simulink model "mariner_simtr"  (R2018b)
settings: Solver=FixedStepAuto  StartTime=0.0  StopTime=600  FixedStep=0.1  RelTol=1e-3
libraries: neural x211, simulink x2
(part 6 of 10)

== system mariner_simtr/NN transform (No normalization)/Layer 4/Delays 1 ==
  "p{4}" : Inport  PortDimensions=24
      mask Display: e = 0.06;c1 = [120 230 180]/255;c2 = ([120 230 180]+0)/(256+128);c3 = ([120 230 180]+128)/(256+128);patch([0 1 1 0],[0 0 1 1],c1);patch([0 1 1 1-e 1-e 0+e],[0 0 1 1-e 0+e 0+e],c2);patch([0 0 1 1-e 0+e 0+e],[0 1 1 1-e 1-e 0+e],c3);plot([0 1 1 0 0],[0 0 1 1 0]);
  mux : Mux  Inputs=1
      mask Display: e = 0.06;c1 = [120 150 230]/255;c2 = ([120 150 230]+0)/383;c3 = ([120 150 230]+128)/383;patch([0 1 1 0],[0 0 1 1],c1);patch([0 1 1 1-e 1-e 0+e],[0 0 1 1-e 0+e 0+e],c2);patch([0 0 1 1-e 0+e 0+e],[0 1 1 1-e 1-e 0+e],c3);plot([0 1 1 0 0],[0 0 1 1 0]);disp('Mux')
  "pd{4,3}" : Outport
      mask Display: e = 0.06;c1 = [120 230 180]/255;c2 = ([120 230 180]+0)/(256+128);c3 = ([120 230 180]+128)/(256+128);patch([0 1 1 0],[0 0 1 1],c1);patch([0 1 1 1-e 1-e 0+e],[0 0 1 1-e 0+e 0+e],c2);patch([0 0 1 1-e 0+e 0+e],[0 1 1 1-e 1-e 0+e],c3);plot([0 1 1 0 0],[0 0 1 1 0]);
  wires:
  mux/1 -> "pd{4,3}"/1
  "p{4}"/1 -> mux/1

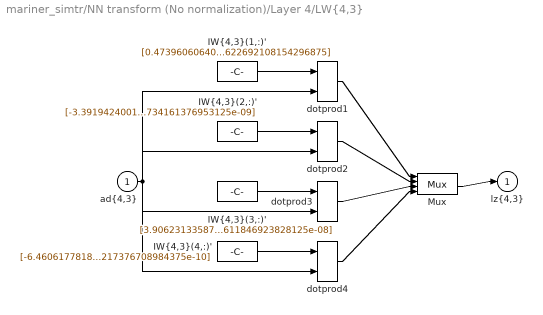
== system mariner_simtr/NN transform (No normalization)/Layer 4/LW{4,3} ==
  "ad{4,3}" : Inport  PortDimensions=24
      mask Display: e = 0.06;c1 = [120 230 180]/255;c2 = ([120 230 180]+0)/(256+128);c3 = ([120 230 180]+128)/(256+128);patch([0 1 1 0],[0 0 1 1],c1);patch([0 1 1 1-e 1-e 0+e],[0 0 1 1-e 0+e 0+e],c2);patch([0 0 1 1-e 0+e 0+e],[0 1 1 1-e 1-e 0+e],c3);plot([0 1 1 0 0],[0 0 1 1 0]);
  "IW{4,3}(1,:)'" : Constant  Value=[0.47396060640014059384128586316364817321300506591796875;0;0;0;0;0.23418587838913584864286576703307218849658966064453125;0.1300136310990274990384563125189743004739284515380859375;0.5442556933540909636093374501797370612621307373046875;0;0;0.1497209490422759803340824191764113493263721466064453125;0.32946160549255931737633318334701471030712127685546875;0;0.58508220152901879718143618447356857359409332275390625;0;0;0.52760521849978292419081071784603409469127655029296875;0;0.4427234693408463872543734396458603441715240478515625;0;0.239017941354947638377126395425875671207904815673828125;0;0;0.342933854164539642095377303121495060622692108154296875]
      mask Display: e = 0.06;c1 = [120 150 230]/255;c2 = ([120 150 230]+0)/383;c3 = ([120 150 230]+128)/383;patch([0 1 1 0],[0 0 1 1],c1);patch([0 1 1 1-e 1-e 0+e],[0 0 1 1-e 0+e 0+e],c2);patch([0 0 1 1-e 0+e 0+e],[0 1 1 1-e 1-e 0+e],c3);plot([0 1 1 0 0],[0 0 1 1 0]);disp('weights');
  "IW{4,3}(2,:)'" : Constant  Value=[-3.391942400136792629749466325699176760810615860464167781174182891845703125e-09;0;0;0;0;-1.6759725826658646329116917372587143575390911109934677369892597198486328125e-09;-9.30453566444665859480412774891629201778897595431772060692310333251953125e-10;-3.89501638174218884460996254154134532665665346939931623637676239013671875e-09;0;0;-1.07149167461716437733348946509913390823243162230937741696834564208984375e-09;-2.35782212547297224439259437540894470686225758981890976428985595703125e-09;0;-4.18719461595151772406936665159825350368549834456644020974636077880859375e-09;0;0;-3.77585503180276468062835277281034940255466381131554953753948211669921875e-09;0;-3.1683907985474438596154613521395371211752944873296655714511871337890625e-09;0;-1.7105539408120519205060434722565597398524772643213509581983089447021484375e-09;0;0;-2.45423722666407805361156200326007426060215266261366195976734161376953125e-09]
      mask Display: e = 0.06;c1 = [120 150 230]/255;c2 = ([120 150 230]+0)/383;c3 = ([120 150 230]+128)/383;patch([0 1 1 0],[0 0 1 1],c1);patch([0 1 1 1-e 1-e 0+e],[0 0 1 1-e 0+e 0+e],c2);patch([0 0 1 1-e 0+e 0+e],[0 1 1 1-e 1-e 0+e],c3);plot([0 1 1 0 0],[0 0 1 1 0]);disp('weights');
  "IW{4,3}(3,:)'" : Constant  Value=[3.906231335871542220591676034847916643144571935408748686313629150390625e-08;0;0;0;0;1.9300849581636230031175206138353839246946108687552623450756072998046875e-08;1.07153259426101197853446330104758288381816555556724779307842254638671875e-08;4.4855791930787298062320773463229617306069485493935644626617431640625e-08;0;0;1.23395187869138592297099253809744556775740420562215149402618408203125e-08;2.715316852794615881804633750716548856729559702216647565364837646484375e-08;0;4.822059002144291084188985961438145277924149922910146415233612060546875e-08;0;0;4.348352813626897564696003575974991850472406440530903637409210205078125e-08;0;3.648785190454878497148385259503389210777868356672115623950958251953125e-08;0;1.9699086591876561340584133740112815491585251947981305420398712158203125e-08;0;0;2.82635142925693801697702611970541841657222903450019657611846923828125e-08]
      mask Display: e = 0.06;c1 = [120 150 230]/255;c2 = ([120 150 230]+0)/383;c3 = ([120 150 230]+128)/383;patch([0 1 1 0],[0 0 1 1],c1);patch([0 1 1 1-e 1-e 0+e],[0 0 1 1-e 0+e 0+e],c2);patch([0 0 1 1-e 0+e 0+e],[0 1 1 1-e 1-e 0+e],c3);plot([0 1 1 0 0],[0 0 1 1 0]);disp('weights');
  "IW{4,3}(4,:)'" : Constant  Value=[-6.460617781862985692955497792739315288113033375339000485837459564208984375e-10;0;0;0;0;-3.19221831670145376018629568929947486199960593467039871029555797576904296875e-10;-1.77227149729209489839184324592546819487903775325321475975215435028076171875e-10;-7.418784716696137475953982663733933533567466156455338932573795318603515625e-10;0;0;-2.0408615668624934789896752164472561175134757149862707592546939849853515625e-10;-4.4909323393439293503977718965253750071919824904398410581052303314208984375e-10;0;-7.9753123374394739103637199349738917675267657614313066005706787109375e-10;0;0;-7.191849801466453163669174789875138120720521328621543943881988525390625e-10;0;-6.0348265919380995223017907338526090443853178157951333560049533843994140625e-10;0;-3.2580723490467324786057817085260963907433762187793035991489887237548828125e-10;0;0;-4.674586797935151118062713950624363634656077692852704785764217376708984375e-10]
      mask Display: e = 0.06;c1 = [120 150 230]/255;c2 = ([120 150 230]+0)/383;c3 = ([120 150 230]+128)/383;patch([0 1 1 0],[0 0 1 1],c1);patch([0 1 1 1-e 1-e 0+e],[0 0 1 1-e 0+e 0+e],c2);patch([0 0 1 1-e 0+e 0+e],[0 1 1 1-e 1-e 0+e],c3);plot([0 1 1 0 0],[0 0 1 1 0]);disp('weights');
  Mux : Mux
      mask Display: e = 0.06;c1 = [120 150 230]/255;c2 = ([120 150 230]+0)/383;c3 = ([120 150 230]+128)/383;patch([0 1 1 0],[0 0 1 1],c1);patch([0 1 1 1-e 1-e 0+e],[0 0 1 1-e 0+e 0+e],c2);patch([0 0 1 1-e 0+e 0+e],[0 1 1 1-e 1-e 0+e],c3);plot([0 1 1 0 0],[0 0 1 1 0]);disp('Mux');
  dotprod{1..4} (4 alike) : neural/Weight Functions/dotprod
  "lz{4,3}" : Outport
      mask Display: e = 0.06;c1 = [120 230 180]/255;c2 = ([120 230 180]+0)/(256+128);c3 = ([120 230 180]+128)/(256+128);patch([0 1 1 0],[0 0 1 1],c1);patch([0 1 1 1-e 1-e 0+e],[0 0 1 1-e 0+e 0+e],c2);patch([0 0 1 1-e 0+e 0+e],[0 1 1 1-e 1-e 0+e],c3);plot([0 1 1 0 0],[0 0 1 1 0]);
  wires:
  Mux/1 -> "lz{4,3}"/1
  dotprod4/1 -> Mux/4
  "IW{4,3}(4,:)'"/1 -> dotprod4/1
  dotprod3/1 -> Mux/3
  "IW{4,3}(3,:)'"/1 -> dotprod3/1
  dotprod2/1 -> Mux/2
  "IW{4,3}(2,:)'"/1 -> dotprod2/1
  dotprod1/1 -> Mux/1
  "ad{4,3}"/1 -> dotprod4/2, dotprod3/2, dotprod2/2, dotprod1/2
  "IW{4,3}(1,:)'"/1 -> dotprod1/1

== system mariner_simtr/NN transform (normalizing)/Layer 1/Delays 1 ==
  "p{1}" : Inport  PortDimensions=7
      mask Display: e = 0.06;c1 = [120 230 180]/255;c2 = ([120 230 180]+0)/(256+128);c3 = ([120 230 180]+128)/(256+128);patch([0 1 1 0],[0 0 1 1],c1);patch([0 1 1 1-e 1-e 0+e],[0 0 1 1-e 0+e 0+e],c2);patch([0 0 1 1-e 0+e 0+e],[0 1 1 1-e 1-e 0+e],c3);plot([0 1 1 0 0],[0 0 1 1 0]);
  mux : Mux  Inputs=1
      mask Display: e = 0.06;c1 = [120 150 230]/255;c2 = ([120 150 230]+0)/383;c3 = ([120 150 230]+128)/383;patch([0 1 1 0],[0 0 1 1],c1);patch([0 1 1 1-e 1-e 0+e],[0 0 1 1-e 0+e 0+e],c2);patch([0 0 1 1-e 0+e 0+e],[0 1 1 1-e 1-e 0+e],c3);plot([0 1 1 0 0],[0 0 1 1 0]);disp('Mux')
  "pd{1,1}" : Outport
      mask Display: e = 0.06;c1 = [120 230 180]/255;c2 = ([120 230 180]+0)/(256+128);c3 = ([120 230 180]+128)/(256+128);patch([0 1 1 0],[0 0 1 1],c1);patch([0 1 1 1-e 1-e 0+e],[0 0 1 1-e 0+e 0+e],c2);patch([0 0 1 1-e 0+e 0+e],[0 1 1 1-e 1-e 0+e],c3);plot([0 1 1 0 0],[0 0 1 1 0]);
  wires:
  mux/1 -> "pd{1,1}"/1
  "p{1}"/1 -> mux/1

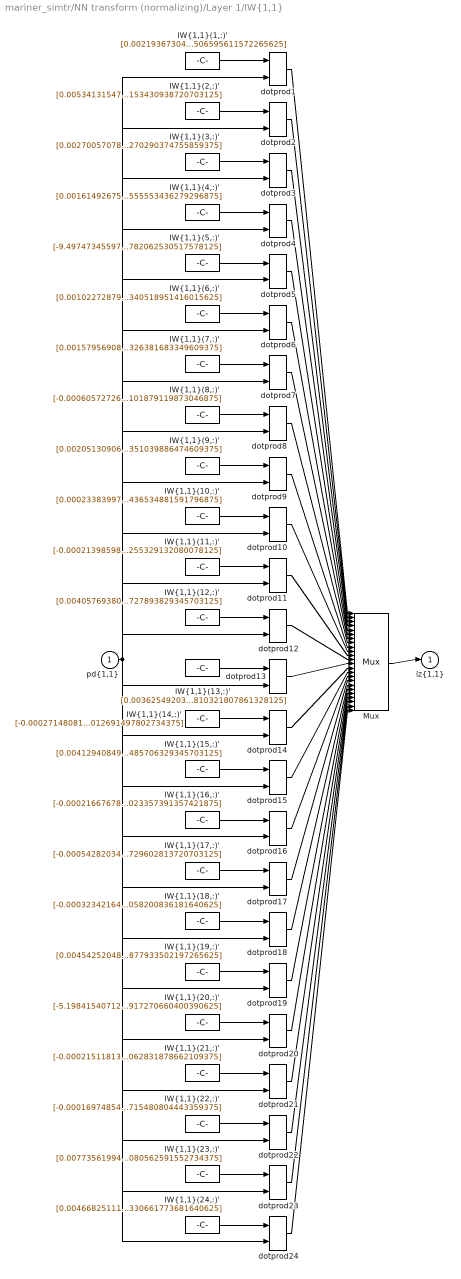
== system mariner_simtr/NN transform (normalizing)/Layer 1/IW{1,1} ==
  "pd{1,1}" : Inport  PortDimensions=7
      mask Display: e = 0.06;c1 = [120 230 180]/255;c2 = ([120 230 180]+0)/(256+128);c3 = ([120 230 180]+128)/(256+128);patch([0 1 1 0],[0 0 1 1],c1);patch([0 1 1 1-e 1-e 0+e],[0 0 1 1-e 0+e 0+e],c2);patch([0 0 1 1-e 0+e 0+e],[0 1 1 1-e 1-e 0+e],c3);plot([0 1 1 0 0],[0 0 1 1 0]);
  "IW{1,1}(1,:)'" : Constant  Value=[0.002193673041712596201435747644836737890727818012237548828125;0.01007863722791245246479530095484733465127646923065185546875;0.06427848875370190118161417558440007269382476806640625;0.009378100723181327647015592674506478942930698394775390625;0.001905390661678683927870991965392022393643856048583984375;0.1275535303877860238142005755435093306005001068115234375;-0.06209769952914169499624819081873283721506595611572265625]
      mask Display: e = 0.06;c1 = [120 150 230]/255;c2 = ([120 150 230]+0)/383;c3 = ([120 150 230]+128)/383;patch([0 1 1 0],[0 0 1 1],c1);patch([0 1 1 1-e 1-e 0+e],[0 0 1 1-e 0+e 0+e],c2);patch([0 0 1 1-e 0+e 0+e],[0 1 1 1-e 1-e 0+e],c3);plot([0 1 1 0 0],[0 0 1 1 0]);disp('Weights');
  "IW{1,1}(10,:)'" : Constant  Value=[0.000233839970507883376273083886331960457027889788150787353515625;0.00132190288831251210634187831516328515135683119297027587890625;0.00836411873984637364853877983250640681944787502288818359375;0.001421281916662076906521239294534098007716238498687744140625;0.0004427467469858896941502235389265251797041855752468109130859375;0.01688283844270412059618280409267754293978214263916015625;-0.00787089206931835920488804703154528397135436534881591796875]
      mask Display: e = 0.06;c1 = [120 150 230]/255;c2 = ([120 150 230]+0)/383;c3 = ([120 150 230]+128)/383;patch([0 1 1 0],[0 0 1 1],c1);patch([0 1 1 1-e 1-e 0+e],[0 0 1 1-e 0+e 0+e],c2);patch([0 0 1 1-e 0+e 0+e],[0 1 1 1-e 1-e 0+e],c3);plot([0 1 1 0 0],[0 0 1 1 0]);disp('Weights');
  "IW{1,1}(11,:)'" : Constant  Value=[-0.00021398598377684005284078694320015756602515466511249542236328125;1.555652484007565269498820671734140574926641420461237430572509765625e-06;-0.000130699675755283832405406752030785355600528419017791748046875;-0.0015584981569765781785064095998905031592585146427154541015625;-0.0014756099760856351832405408686099690385162830352783203125;-0.00276861067318717561647201108598892460577189922332763671875;-0.0006140065643789297152033146431904242490418255329132080078125]
      mask Display: e = 0.06;c1 = [120 150 230]/255;c2 = ([120 150 230]+0)/383;c3 = ([120 150 230]+128)/383;patch([0 1 1 0],[0 0 1 1],c1);patch([0 1 1 1-e 1-e 0+e],[0 0 1 1-e 0+e 0+e],c2);patch([0 0 1 1-e 0+e 0+e],[0 1 1 1-e 1-e 0+e],c3);plot([0 1 1 0 0],[0 0 1 1 0]);disp('Weights');
  "IW{1,1}(12,:)'" : Constant  Value=[0.004057693800549562641866163659187805023975670337677001953125;0.00968990318378684135913747610402424470521509647369384765625;0.04410311055866979190742682703785249032080173492431640625;0.0002607289566118379761129608684910863303230144083499908447265625;-0.004837126710472833095166844685763862798921763896942138671875;0.08180429634076540057474602463116752915084362030029296875;-0.053530711199899994046091933341813273727893829345703125]
      mask Display: e = 0.06;c1 = [120 150 230]/255;c2 = ([120 150 230]+0)/383;c3 = ([120 150 230]+128)/383;patch([0 1 1 0],[0 0 1 1],c1);patch([0 1 1 1-e 1-e 0+e],[0 0 1 1-e 0+e 0+e],c2);patch([0 0 1 1-e 0+e 0+e],[0 1 1 1-e 1-e 0+e],c3);plot([0 1 1 0 0],[0 0 1 1 0]);disp('Weights');
  "IW{1,1}(13,:)'" : Constant  Value=[0.0036254920367055870449035648306335133383981883525848388671875;0.010664121247743872655799890480921021662652492523193359375;0.0556958079923742521710749997509992681443691253662109375;0.00407235777173577638554657909253364778123795986175537109375;-0.0023858881292989834836670848261519495281390845775604248046875;0.10682129809699743294704177287712809629738330841064453125;-0.061128103385034777972339981033655931241810321807861328125]
      mask Display: e = 0.06;c1 = [120 150 230]/255;c2 = ([120 150 230]+0)/383;c3 = ([120 150 230]+128)/383;patch([0 1 1 0],[0 0 1 1],c1);patch([0 1 1 1-e 1-e 0+e],[0 0 1 1-e 0+e 0+e],c2);patch([0 0 1 1-e 0+e 0+e],[0 1 1 1-e 1-e 0+e],c3);plot([0 1 1 0 0],[0 0 1 1 0]);disp('Weights');
  "IW{1,1}(14,:)'" : Constant  Value=[-0.0002714808174996637710023328349251414692844264209270477294921875;1.97363304192348819730991847654077986362608498893678188323974609375e-06;-0.00016581672404294183951166397061882662455900572240352630615234375;-0.0019772433047244276048404199030983363627456128597259521484375;-0.001872084309204442853502570187629316933453083038330078125;-0.0035124949570474691719346171936422251746989786624908447265625;-0.000778980945880768430554519365927035323693417012691497802734375]
      mask Display: e = 0.06;c1 = [120 150 230]/255;c2 = ([120 150 230]+0)/383;c3 = ([120 150 230]+128)/383;patch([0 1 1 0],[0 0 1 1],c1);patch([0 1 1 1-e 1-e 0+e],[0 0 1 1-e 0+e 0+e],c2);patch([0 0 1 1-e 0+e 0+e],[0 1 1 1-e 1-e 0+e],c3);plot([0 1 1 0 0],[0 0 1 1 0]);disp('Weights');
  "IW{1,1}(15,:)'" : Constant  Value=[0.00412940849085605653223662869777399464510381221771240234375;0.0125144097935502053575707037680331268347799777984619140625;0.06657084630720487561372777918222709558904170989990234375;0.005343971815902463957936863181430453551001846790313720703125;-0.002375175811461496290510897466674578026868402957916259765625;0.1280752735319928004020795242468011565506458282470703125;-0.07216621163924659410060513664575410075485706329345703125]
      mask Display: e = 0.06;c1 = [120 150 230]/255;c2 = ([120 150 230]+0)/383;c3 = ([120 150 230]+128)/383;patch([0 1 1 0],[0 0 1 1],c1);patch([0 1 1 1-e 1-e 0+e],[0 0 1 1-e 0+e 0+e],c2);patch([0 0 1 1-e 0+e 0+e],[0 1 1 1-e 1-e 0+e],c3);plot([0 1 1 0 0],[0 0 1 1 0]);disp('Weights');
  "IW{1,1}(16,:)'" : Constant  Value=[-0.0002166767824471827938968837568012304473086260259151458740234375;1.5752142681597100263234632888664776828591129742562770843505859375e-06;-0.0001323431783227408948915015951541818139958195388317108154296875;-0.00157809572451108985624568248340438003651797771453857421875;-0.00149416525382624018093713491595053710625506937503814697265625;-0.00280342498105252795059794124199470388703048229217529296875;-0.0006217274815055631558002868786161343450658023357391357421875]
      mask Display: e = 0.06;c1 = [120 150 230]/255;c2 = ([120 150 230]+0)/383;c3 = ([120 150 230]+128)/383;patch([0 1 1 0],[0 0 1 1],c1);patch([0 1 1 1-e 1-e 0+e],[0 0 1 1-e 0+e 0+e],c2);patch([0 0 1 1-e 0+e 0+e],[0 1 1 1-e 1-e 0+e],c3);plot([0 1 1 0 0],[0 0 1 1 0]);disp('Weights');
  "IW{1,1}(17,:)'" : Constant  Value=[-0.000542820340012894748775440501020739247906021773815155029296875;0.0011180280954363225505432399842220547725446522235870361328125;0.01445126669371987228329690111650052131153643131256103515625;0.004532129827479853927119091139275042223744094371795654296875;0.0028409244258676695678300649916536713135428726673126220703125;0.0309138346973172571663379670781068853102624416351318359375;-0.00952122896890898913480061338532323134131729602813720703125]
      mask Display: e = 0.06;c1 = [120 150 230]/255;c2 = ([120 150 230]+0)/383;c3 = ([120 150 230]+128)/383;patch([0 1 1 0],[0 0 1 1],c1);patch([0 1 1 1-e 1-e 0+e],[0 0 1 1-e 0+e 0+e],c2);patch([0 0 1 1-e 0+e 0+e],[0 1 1 1-e 1-e 0+e],c3);plot([0 1 1 0 0],[0 0 1 1 0]);disp('Weights');
  "IW{1,1}(18,:)'" : Constant  Value=[-0.00032342164775511490597270647384675612556748092174530029296875;2.35123665960109029350664881785615278886325540952384471893310546875e-06;-0.0001975414639209283908759251513487242846167646348476409912109375;-0.002355537652775906674873507284928564331494271755218505859375;-0.0022302592042999021433591355645376097527332603931427001953125;-0.004184519986357389254028049663247657008469104766845703125;-0.000928018794871073222398083490958242691704072058200836181640625]
      mask Display: e = 0.06;c1 = [120 150 230]/255;c2 = ([120 150 230]+0)/383;c3 = ([120 150 230]+128)/383;patch([0 1 1 0],[0 0 1 1],c1);patch([0 1 1 1-e 1-e 0+e],[0 0 1 1-e 0+e 0+e],c2);patch([0 0 1 1-e 0+e 0+e],[0 1 1 1-e 1-e 0+e],c3);plot([0 1 1 0 0],[0 0 1 1 0]);disp('Weights');
  "IW{1,1}(19,:)'" : Constant  Value=[0.004542520485955059590665872093495636363513767719268798828125;0.0103951453252636195900837634553681709803640842437744140625;0.04474717113630999332229976062080822885036468505859375;-0.00068324257684836109914827684264082563458941876888275146484375;-0.005860426026166591639832148530331323854625225067138671875;0.082300379739235596243673853678046725690364837646484375;-0.0561881360524382478249805217274115420877933502197265625]
      mask Display: e = 0.06;c1 = [120 150 230]/255;c2 = ([120 150 230]+0)/383;c3 = ([120 150 230]+128)/383;patch([0 1 1 0],[0 0 1 1],c1);patch([0 1 1 1-e 1-e 0+e],[0 0 1 1-e 0+e 0+e],c2);patch([0 0 1 1-e 0+e 0+e],[0 1 1 1-e 1-e 0+e],c3);plot([0 1 1 0 0],[0 0 1 1 0]);disp('Weights');
  "IW{1,1}(2,:)'" : Constant  Value=[0.005341315471311857722425120442721890867687761783599853515625;0.00786487089126441767106268088127762894146144390106201171875;0.0159297582403710204224100976944100693799555301666259765625;-0.00906848666534805329664248318977115559391677379608154296875;-0.010860874477614530786429014597160858102142810821533203125;0.0209759870627989723768092034106302889995276927947998046875;-0.035642312701089536031151538963968050666153430938720703125]
      mask Display: e = 0.06;c1 = [120 150 230]/255;c2 = ([120 150 230]+0)/383;c3 = ([120 150 230]+128)/383;patch([0 1 1 0],[0 0 1 1],c1);patch([0 1 1 1-e 1-e 0+e],[0 0 1 1-e 0+e 0+e],c2);patch([0 0 1 1-e 0+e 0+e],[0 1 1 1-e 1-e 0+e],c3);plot([0 1 1 0 0],[0 0 1 1 0]);disp('Weights');
  "IW{1,1}(20,:)'" : Constant  Value=[-5.19841540712387745648732917391754426716943271458148956298828125e-05;3.779185766327267902763638492136255564446400967426598072052001953125e-07;-3.17512014647136129696751438711288528793375007808208465576171875e-05;-0.0003786098831431052697503447657112474189489148557186126708984375;-0.0003584736485633053235978773276571018868708051741123199462890625;-0.000672585564988842561119641860756246387609280645847320556640625;-0.00014916216137180038207345200707010235419147647917270660400390625]
      mask Display: e = 0.06;c1 = [120 150 230]/255;c2 = ([120 150 230]+0)/383;c3 = ([120 150 230]+128)/383;patch([0 1 1 0],[0 0 1 1],c1);patch([0 1 1 1-e 1-e 0+e],[0 0 1 1-e 0+e 0+e],c2);patch([0 0 1 1-e 0+e 0+e],[0 1 1 1-e 1-e 0+e],c3);plot([0 1 1 0 0],[0 0 1 1 0]);disp('Weights');
  "IW{1,1}(21,:)'" : Constant  Value=[-0.00021511813712368830879551051538101091864518821239471435546875;1.563883103250626863245224297538360502812793129123747348785400390625e-06;-0.0001313911793422287469478015875523624345078133046627044677734375;-0.0015667438321059373208810061584017603308893740177154541015625;-0.0014834171078592279548191701366022243746556341648101806640625;-0.0027832587907153229049572740194662401336245238780975341796875;-0.0006172551397041494379569481765201999223791062831878662109375]
      mask Display: e = 0.06;c1 = [120 150 230]/255;c2 = ([120 150 230]+0)/383;c3 = ([120 150 230]+128)/383;patch([0 1 1 0],[0 0 1 1],c1);patch([0 1 1 1-e 1-e 0+e],[0 0 1 1-e 0+e 0+e],c2);patch([0 0 1 1-e 0+e 0+e],[0 1 1 1-e 1-e 0+e],c3);plot([0 1 1 0 0],[0 0 1 1 0]);disp('Weights');
  "IW{1,1}(22,:)'" : Constant  Value=[-0.0001697485419579625588563931426477893182891421020030975341796875;1.234051577987989783413160481406745105914524174295365810394287109375e-06;-0.000103680058862972747368846881954596028663218021392822265625;-0.0012363089634262747207316124331555329263210296630859375;-0.001170556302418099790807470839126835926435887813568115234375;-0.00219625424398268986880822239982080645859241485595703125;-0.000487072644742064602384201688067832947126589715480804443359375]
      mask Display: e = 0.06;c1 = [120 150 230]/255;c2 = ([120 150 230]+0)/383;c3 = ([120 150 230]+128)/383;patch([0 1 1 0],[0 0 1 1],c1);patch([0 1 1 1-e 1-e 0+e],[0 0 1 1-e 0+e 0+e],c2);patch([0 0 1 1-e 0+e 0+e],[0 1 1 1-e 1-e 0+e],c3);plot([0 1 1 0 0],[0 0 1 1 0]);disp('Weights');
  "IW{1,1}(23,:)'" : Constant  Value=[0.0077356199402919371965747785679923254065215587615966796875;0.0107666319110372825373911354063238832168281078338623046875;0.0141533294909642511083536220439782482571899890899658203125;-0.01195949879128527758298528027580687194131314754486083984375;-0.01350610700416236646670409271564494702033698558807373046875;0.014607374015862768790174897048927959986031055450439453125;-0.038138613941220277092636337101794197224080562591552734375]
      mask Display: e = 0.06;c1 = [120 150 230]/255;c2 = ([120 150 230]+0)/383;c3 = ([120 150 230]+128)/383;patch([0 1 1 0],[0 0 1 1],c1);patch([0 1 1 1-e 1-e 0+e],[0 0 1 1-e 0+e 0+e],c2);patch([0 0 1 1-e 0+e 0+e],[0 1 1 1-e 1-e 0+e],c3);plot([0 1 1 0 0],[0 0 1 1 0]);disp('Weights');
  "IW{1,1}(24,:)'" : Constant  Value=[0.004668251115044565018041833326378764468245208263397216796875;0.0110530901300454863223077239808844751678407192230224609375;0.04953707673890277163319950659570167772471904754638671875;2.8616292833680574540268504168949448285275138914585113525390625e-05;-0.00570425961346450287325904326962699997238814830780029296875;0.091793169641070371245206160892848856747150421142578125;-0.060688048887842273304560336555368849076330661773681640625]
      mask Display: e = 0.06;c1 = [120 150 230]/255;c2 = ([120 150 230]+0)/383;c3 = ([120 150 230]+128)/383;patch([0 1 1 0],[0 0 1 1],c1);patch([0 1 1 1-e 1-e 0+e],[0 0 1 1-e 0+e 0+e],c2);patch([0 0 1 1-e 0+e 0+e],[0 1 1 1-e 1-e 0+e],c3);plot([0 1 1 0 0],[0 0 1 1 0]);disp('Weights');
  "IW{1,1}(3,:)'" : Constant  Value=[0.0027005707852823909904949051252742719952948391437530517578125;0.005405671334519438105126187821269923006184399127960205078125;0.0205483837030053552441533071259982534684240818023681640625;-0.00182621366635711546155818041370366699993610382080078125;-0.0041885196127235575780378695753825013525784015655517578125;0.0362459124173357960518870868327212519943714141845703125;-0.028301495848097178720248479066867730580270290374755859375]
      mask Display: e = 0.06;c1 = [120 150 230]/255;c2 = ([120 150 230]+0)/383;c3 = ([120 150 230]+128)/383;patch([0 1 1 0],[0 0 1 1],c1);patch([0 1 1 1-e 1-e 0+e],[0 0 1 1-e 0+e 0+e],c2);patch([0 0 1 1-e 0+e 0+e],[0 1 1 1-e 1-e 0+e],c3);plot([0 1 1 0 0],[0 0 1 1 0]);disp('Weights');
  "IW{1,1}(4,:)'" : Constant  Value=[0.00161492675644769466576644578736932089668698608875274658203125;0.005002810647706273060320025791725129238329827785491943359375;0.026905449958142667321592256257645203731954097747802734375;0.0021265505848762906830617946951633712160401046276092529296875;-0.0010026758149205999316733173287730096490122377872467041015625;0.051912214616385989052194105397575185634195804595947265625;-0.0291269375598666273308179341938739526085555553436279296875]
      mask Display: e = 0.06;c1 = [120 150 230]/255;c2 = ([120 150 230]+0)/383;c3 = ([120 150 230]+128)/383;patch([0 1 1 0],[0 0 1 1],c1);patch([0 1 1 1-e 1-e 0+e],[0 0 1 1-e 0+e 0+e],c2);patch([0 0 1 1-e 0+e 0+e],[0 1 1 1-e 1-e 0+e],c3);plot([0 1 1 0 0],[0 0 1 1 0]);disp('Weights');
  "IW{1,1}(5,:)'" : Constant  Value=[-9.4974734559713202002202703244648773761582560837268829345703125e-05;6.90454950015457982290148324089340547971005435101687908172607421875e-07;-5.8009252722108261613766233555367080043652094900608062744140625e-05;-0.0006917179628223167793532599745276456815190613269805908203125;-0.000654929184233599896540478635387216854724101722240447998046875;-0.001228809752602076123262353490872555994428694248199462890625;-0.0002725183651777006552281712448149164629285223782062530517578125]
      mask Display: e = 0.06;c1 = [120 150 230]/255;c2 = ([120 150 230]+0)/383;c3 = ([120 150 230]+128)/383;patch([0 1 1 0],[0 0 1 1],c1);patch([0 1 1 1-e 1-e 0+e],[0 0 1 1-e 0+e 0+e],c2);patch([0 0 1 1-e 0+e 0+e],[0 1 1 1-e 1-e 0+e],c3);plot([0 1 1 0 0],[0 0 1 1 0]);disp('Weights');
  "IW{1,1}(6,:)'" : Constant  Value=[0.00102272879663423284755940922963191042072139680385589599609375;0.0034883131651030113880296301687167215277440845966339111328125;0.019293611832004446682287124303911696188151836395263671875;0.002109357050699957325523570261793793179094791412353515625;-0.0001317295247622174837569264393977164218085817992687225341796875;0.037662512423869830280320769588797702454030513763427734375;-0.0200624484715146746138803024450680823065340518951416015625]
      mask Display: e = 0.06;c1 = [120 150 230]/255;c2 = ([120 150 230]+0)/383;c3 = ([120 150 230]+128)/383;patch([0 1 1 0],[0 0 1 1],c1);patch([0 1 1 1-e 1-e 0+e],[0 0 1 1-e 0+e 0+e],c2);patch([0 0 1 1-e 0+e 0+e],[0 1 1 1-e 1-e 0+e],c3);plot([0 1 1 0 0],[0 0 1 1 0]);disp('Weights');
  "IW{1,1}(7,:)'" : Constant  Value=[0.001579569084618971837319367779173262533731758594512939453125;0.0047880506841537530393626553859576233662664890289306640625;0.0251968055972473480019768743431995972059667110443115234375;0.0020211764530174186789424073396048697759397327899932861328125;-0.0009042296406198148915611678688719621277414262294769287109375;0.048545282615784814128634394592154421843588352203369140625;-0.027394576442071903732422555322045809589326381683349609375]
      mask Display: e = 0.06;c1 = [120 150 230]/255;c2 = ([120 150 230]+0)/383;c3 = ([120 150 230]+128)/383;patch([0 1 1 0],[0 0 1 1],c1);patch([0 1 1 1-e 1-e 0+e],[0 0 1 1-e 0+e 0+e],c2);patch([0 0 1 1-e 0+e 0+e],[0 1 1 1-e 1-e 0+e],c3);plot([0 1 1 0 0],[0 0 1 1 0]);disp('Weights');
  "IW{1,1}(8,:)'" : Constant  Value=[-0.000605727261060985135675271973099142996943555772304534912109375;0.00411159823386174350101640584398410283029079437255859375;0.0397296835213906407435757728308090008795261383056640625;0.01060868503206854364384614797245376394130289554595947265625;0.0059633048316824234513777724941974156536161899566650390625;0.08336232145569417995023542289345641620457172393798828125;-0.0299056293533108696891531508299522101879119873046875]
      mask Display: e = 0.06;c1 = [120 150 230]/255;c2 = ([120 150 230]+0)/383;c3 = ([120 150 230]+128)/383;patch([0 1 1 0],[0 0 1 1],c1);patch([0 1 1 1-e 1-e 0+e],[0 0 1 1-e 0+e 0+e],c2);patch([0 0 1 1-e 0+e 0+e],[0 1 1 1-e 1-e 0+e],c3);plot([0 1 1 0 0],[0 0 1 1 0]);disp('Weights');
  "IW{1,1}(9,:)'" : Constant  Value=[0.002051309064835260716208598097409776528365910053253173828125;0.00482129619121732071185260082302193040959537029266357421875;-0.000577839024632721015052594371042005150229670107364654541015625;-0.007392359173643552917865040541300913901068270206451416015625;-0.006917013580534855064774202304533901042304933071136474609375;-0.01477191790259893382220024449225093121640384197235107421875;-0.01006430030162162869711295343222445808351039886474609375]
      mask Display: e = 0.06;c1 = [120 150 230]/255;c2 = ([120 150 230]+0)/383;c3 = ([120 150 230]+128)/383;patch([0 1 1 0],[0 0 1 1],c1);patch([0 1 1 1-e 1-e 0+e],[0 0 1 1-e 0+e 0+e],c2);patch([0 0 1 1-e 0+e 0+e],[0 1 1 1-e 1-e 0+e],c3);plot([0 1 1 0 0],[0 0 1 1 0]);disp('Weights');
  Mux : Mux  Inputs=24
      mask Display: e = 0.06;c1 = [120 150 230]/255;c2 = ([120 150 230]+0)/383;c3 = ([120 150 230]+128)/383;patch([0 1 1 0],[0 0 1 1],c1);patch([0 1 1 1-e 1-e 0+e],[0 0 1 1-e 0+e 0+e],c2);patch([0 0 1 1-e 0+e 0+e],[0 1 1 1-e 1-e 0+e],c3);plot([0 1 1 0 0],[0 0 1 1 0]);disp('Mux');
  dotprod{1..24} (24 alike) : neural/Weight Functions/dotprod
  "iz{1,1}" : Outport
      mask Display: e = 0.06;c1 = [120 230 180]/255;c2 = ([120 230 180]+0)/(256+128);c3 = ([120 230 180]+128)/(256+128);patch([0 1 1 0],[0 0 1 1],c1);patch([0 1 1 1-e 1-e 0+e],[0 0 1 1-e 0+e 0+e],c2);patch([0 0 1 1-e 0+e 0+e],[0 1 1 1-e 1-e 0+e],c3);plot([0 1 1 0 0],[0 0 1 1 0]);
  wires:
  Mux/1 -> "iz{1,1}"/1
  dotprod24/1 -> Mux/24
  "IW{1,1}(24,:)'"/1 -> dotprod24/1
  dotprod23/1 -> Mux/23
  "IW{1,1}(23,:)'"/1 -> dotprod23/1
  dotprod22/1 -> Mux/22
  "IW{1,1}(22,:)'"/1 -> dotprod22/1
  dotprod21/1 -> Mux/21
  "IW{1,1}(21,:)'"/1 -> dotprod21/1
  dotprod20/1 -> Mux/20
  "IW{1,1}(20,:)'"/1 -> dotprod20/1
  dotprod19/1 -> Mux/19
  "IW{1,1}(19,:)'"/1 -> dotprod19/1
  dotprod18/1 -> Mux/18
  "IW{1,1}(18,:)'"/1 -> dotprod18/1
  dotprod17/1 -> Mux/17
  "IW{1,1}(17,:)'"/1 -> dotprod17/1
  dotprod16/1 -> Mux/16
  "IW{1,1}(16,:)'"/1 -> dotprod16/1
  dotprod15/1 -> Mux/15
  "IW{1,1}(15,:)'"/1 -> dotprod15/1
  dotprod14/1 -> Mux/14
  "IW{1,1}(14,:)'"/1 -> dotprod14/1
  dotprod13/1 -> Mux/13
  "IW{1,1}(13,:)'"/1 -> dotprod13/1
  dotprod12/1 -> Mux/12
  "IW{1,1}(12,:)'"/1 -> dotprod12/1
  dotprod11/1 -> Mux/11
  "IW{1,1}(11,:)'"/1 -> dotprod11/1
  dotprod10/1 -> Mux/10
  "IW{1,1}(10,:)'"/1 -> dotprod10/1
  dotprod9/1 -> Mux/9
  "IW{1,1}(9,:)'"/1 -> dotprod9/1
  dotprod8/1 -> Mux/8
  "IW{1,1}(8,:)'"/1 -> dotprod8/1
  dotprod7/1 -> Mux/7
  "IW{1,1}(7,:)'"/1 -> dotprod7/1
  dotprod6/1 -> Mux/6
  "IW{1,1}(6,:)'"/1 -> dotprod6/1
  dotprod5/1 -> Mux/5
  "IW{1,1}(5,:)'"/1 -> dotprod5/1
  dotprod4/1 -> Mux/4
  "IW{1,1}(4,:)'"/1 -> dotprod4/1
  dotprod3/1 -> Mux/3
  "IW{1,1}(3,:)'"/1 -> dotprod3/1
  dotprod2/1 -> Mux/2
  "IW{1,1}(2,:)'"/1 -> dotprod2/1
  dotprod1/1 -> Mux/1
  "pd{1,1}"/1 -> dotprod24/2, dotprod23/2, dotprod22/2, dotprod21/2, dotprod20/2, dotprod19/2, dotprod18/2, dotprod17/2, dotprod16/2, dotprod15/2, dotprod14/2, dotprod13/2, dotprod12/2, dotprod11/2, dotprod10/2, dotprod9/2, dotprod8/2, dotprod7/2, dotprod6/2, dotprod5/2, dotprod4/2, dotprod3/2, dotprod2/2, dotprod1/2
  "IW{1,1}(1,:)'"/1 -> dotprod1/1

== system mariner_simtr/NN transform (normalizing)/Layer 2/Delays 1 ==
  "p{2}" : Inport  PortDimensions=24
      mask Display: e = 0.06;c1 = [120 230 180]/255;c2 = ([120 230 180]+0)/(256+128);c3 = ([120 230 180]+128)/(256+128);patch([0 1 1 0],[0 0 1 1],c1);patch([0 1 1 1-e 1-e 0+e],[0 0 1 1-e 0+e 0+e],c2);patch([0 0 1 1-e 0+e 0+e],[0 1 1 1-e 1-e 0+e],c3);plot([0 1 1 0 0],[0 0 1 1 0]);
  mux : Mux  Inputs=1
      mask Display: e = 0.06;c1 = [120 150 230]/255;c2 = ([120 150 230]+0)/383;c3 = ([120 150 230]+128)/383;patch([0 1 1 0],[0 0 1 1],c1);patch([0 1 1 1-e 1-e 0+e],[0 0 1 1-e 0+e 0+e],c2);patch([0 0 1 1-e 0+e 0+e],[0 1 1 1-e 1-e 0+e],c3);plot([0 1 1 0 0],[0 0 1 1 0]);disp('Mux')
  "pd{2,1}" : Outport
      mask Display: e = 0.06;c1 = [120 230 180]/255;c2 = ([120 230 180]+0)/(256+128);c3 = ([120 230 180]+128)/(256+128);patch([0 1 1 0],[0 0 1 1],c1);patch([0 1 1 1-e 1-e 0+e],[0 0 1 1-e 0+e 0+e],c2);patch([0 0 1 1-e 0+e 0+e],[0 1 1 1-e 1-e 0+e],c3);plot([0 1 1 0 0],[0 0 1 1 0]);
  wires:
  mux/1 -> "pd{2,1}"/1
  "p{2}"/1 -> mux/1
